simulink model "ABS_contDyn_model"  (R2022b)
settings: Solver=VariableStepAuto  StartTime=0.0  StopTime=tf  FixedStep=dt  MaxStep=dt  RelTol=1e-3
values from neighbouring files (symbols this model uses):
  hv = 0.3    [mainABS.m]
  init_speed = 100    [mainABS.m]
  lambda1_th = 0.2    [mainABS.m]
  lambda2_th = 0.1    [mainABS.m]
  omega_act = 70    [mainABS.m]
  omega_LPF = 100    [mainABS.m]
  rho = 0.9    [mainABS.m]
  rho_off = 0.9    [mainABS.m]
  rho_on = 1.1    [mainABS.m]
  tau_delay = 10e-3    (= 0.01)    [mainABS.m]
  Tb_dot_max = k    (= 5000)    [mainABS.m]
  Tb_max = 1500    [mainABS.m]
  v_on = 2.5    [mainABS.m]
  v_stop = 0.1    [mainABS.m]
undefined symbols (not defined in the file or in its folder): auxdata
libraries: simulink x2, dspsigops x1
settings Model: Creator=luca  LastModifiedBy=giacomo
settings SolverCC: AlgebraicLoopSolver=TrustRegion
settings DataIOCC: LimitDataPoints=on  ReturnWorkspaceOutputs=off
settings OptimizationCC: LifeSpan=inf
settings DebuggingCC: UnconnectedInputMsg=warning  UnconnectedOutputMsg=warning  UnconnectedLineMsg=warning  AllowSymbolicDim=off  SFUnexpectedBacktrackingDiag=warning  SFNoUnconditionalDefaultTransitionDiag=warning  SFExecutionAtInitializationDiag=none  SFMachineParentedDataDiag=warning  ArithmeticOperatorsInVariantConditions=warning
settings ModelReferenceCC: EnableRefExpFcnMdlSchedulingChecks=on  PropagateSignalLabelsOutOfModel=off
settings SFSimCC: SimUseLocalCustomCode=off  CustomCodeUndefinedFunction=UseInterfaceOnly
settings RTWCC: RTWUseLocalCustomCode=off
settings CodeAppCC: StateflowObjectComments=on
settings GRTTargetCC: TargetLangStandard=C89/C90 (ANSI)
settings ConfigComp: CovMetricSettings=dw  CovSaveCumulativeToWorkspaceVar=on  CovSaveSingleToWorkspaceVar=on  CovExternalEMLEnable=off

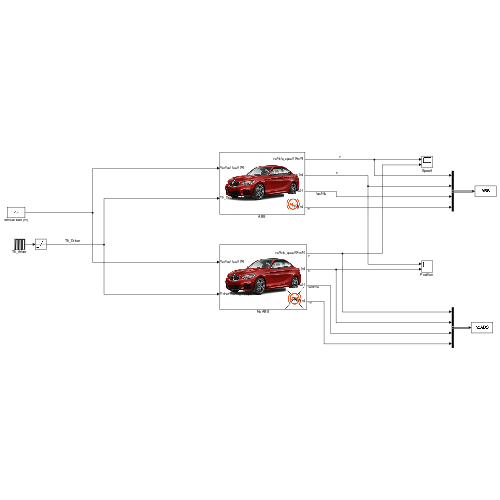
[thumbnail: Simulink's stored preview of the top-level diagram]
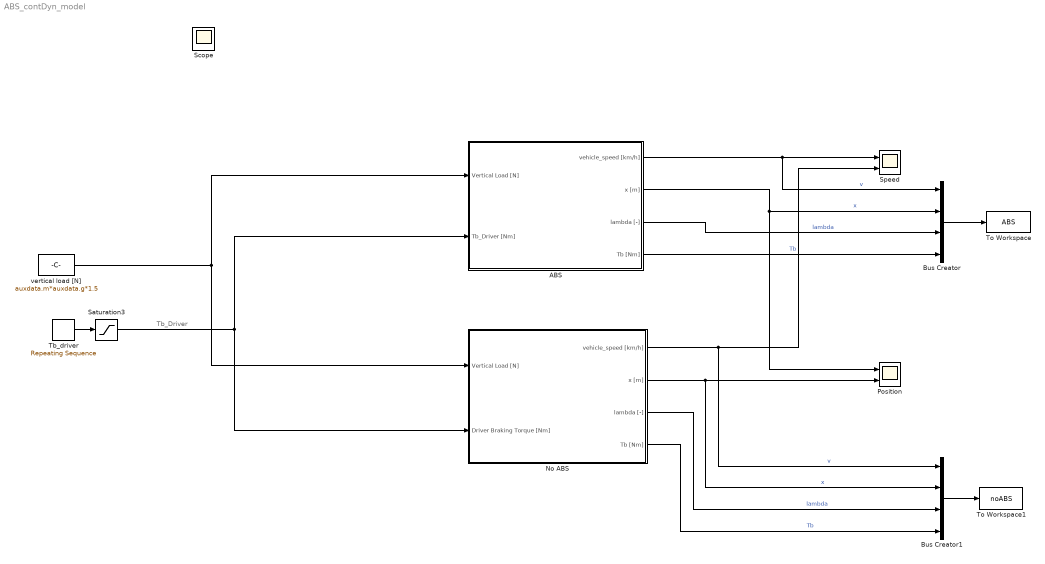
== system ABS_contDyn_model ==
  note: Tb_Driver
  ABS : Subsystem
      mask Display: image('figures/ABScar_on.png');
  Bus Creator : BusCreator  Inputs=4
  Bus Creator1 : BusCreator  Inputs=4
  No ABS : Subsystem
      mask Display: image('figures/ABS_off.png');
  Position : Scope  NumInputPorts=2
  Saturation3 : Saturate  UpperLimit=Tb_max  LowerLimit=0
  Speed : Scope  NumInputPorts=2
  Tb_driver : simulink/Sources/Repeating Sequence  rep_seq_t=time_manoeuvre  rep_seq_y=output_manoeuvre
  To Workspace : ToWorkspace  VariableName=ABS  SaveFormat=Timeseries  SampleTime=-1
  To Workspace1 : ToWorkspace  VariableName=noABS  SaveFormat=Timeseries  SampleTime=-1
  vertical load [N] : Constant  Value=auxdata.m*auxdata.g*1.5
  Scope : Scope
  wires:
  vertical load [N]/1 -> No ABS/1(Vertical Load [N]), ABS/1(Vertical Load [N])
  Saturation3/1 -> No ABS/2(Driver Braking Torque [Nm]), ABS/2(Tb_Driver [Nm])
  No ABS/1(" vehicle_speed [km/h]") -> Speed/2, Bus Creator1/1  "v"
  No ABS/2(x [m]) -> Position/2, Bus Creator1/2  "x"
  ABS/1(vehicle_speed [km/h]) -> Bus Creator/1, Speed/1  "v"
  ABS/2(x [m]) -> Position/1, Bus Creator/2  "x"
  Bus Creator/1 -> To Workspace/1
  ABS/3(lambda [-]) -> Bus Creator/3  "lambda"
  ABS/4(Tb [Nm]) -> Bus Creator/4  "Tb"
  Bus Creator1/1 -> To Workspace1/1
  No ABS/3(lambda [-]) -> Bus Creator1/3  "lambda"
  No ABS/4(Tb [Nm]) -> Bus Creator1/4  "Tb"
  Tb_driver/1 -> Saturation3/1

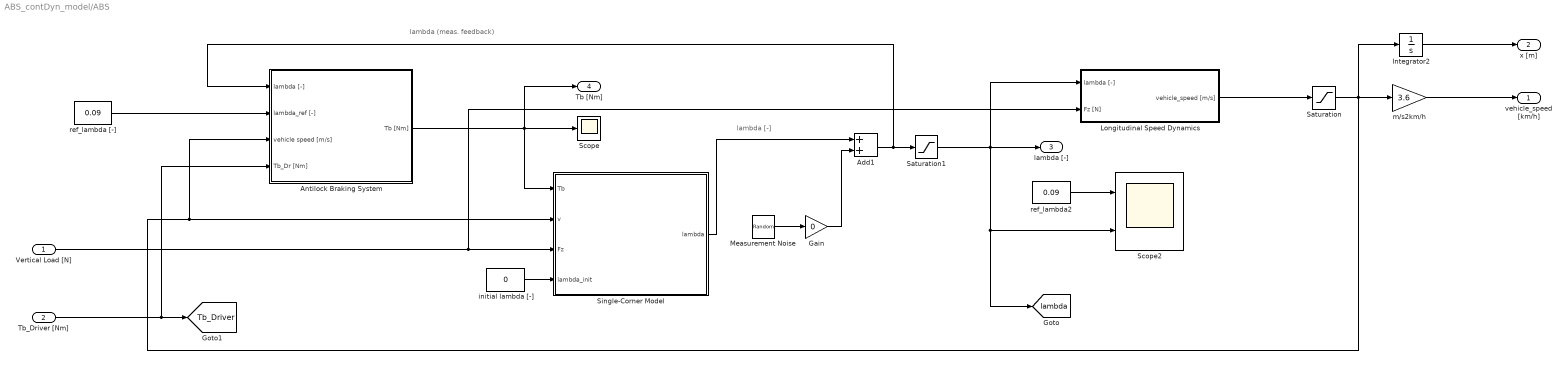
== system ABS_contDyn_model/ABS ==
  note: lambda [-]
  note: lambda (meas. feedback)
  Vertical Load [N] : Inport
  Tb_Driver [Nm] : Inport  Port=2
  Add1 : Sum
  Antilock Braking System : Subsystem
      mask Display: image('figures/ABS_on.png');
  Gain : Gain  Gain=0
  Integrator2 : Integrator
  Longitudinal Speed Dynamics : Subsystem
  Measurement Noise : RandomNumber  Variance=2e-5  SampleTime=0.001
  Saturation : Saturate  UpperLimit=100  LowerLimit=1e-3
  Saturation1 : Saturate  UpperLimit=1  LowerLimit=0
  Scope : Scope
  Scope2 : Scope  NumInputPorts=2
  Single-Corner Model : Subsystem
      mask Display:
      | image('figures/caliper_img.jpeg');
      | color('red');
      | port_label('output',1,'lambda');
      | port_label('input',1,'Tb');
      | port_label('input',2,'v');
      | port_label('input',3,'Fz');
      | port_label('input',4,'lambda_init');
  initial lambda [-] : Constant  Value=0
  m/s2km/h : Gain  Gain=3.6
  ref_lambda [-] : Constant  Value=0.09
  ref_lambda2 : Constant  Value=0.09
  vehicle_speed [km/h] : Outport
  x [m] : Outport  Port=2
  lambda [-] : Outport  Port=3
  Tb [Nm] : Outport  Port=4
  tag scope: Tb_Driver=global, lambda=global
  wires:
  m/s2km/h/1 -> vehicle_speed [km/h]/1
  Integrator2/1 -> x [m]/1
  Longitudinal Speed Dynamics/1(vehicle_speed [m/s]) -> Saturation/1
  Antilock Braking System/1(Tb [Nm]) -> Tb [Nm]/1, Single-Corner Model/1(Tb), Scope/1
  Saturation1/1 -> lambda [-]/1, Scope2/2, [lambda], Longitudinal Speed Dynamics/1(lambda [-])
  ref_lambda [-]/1 -> Antilock Braking System/2(lambda_ref [-])
  Gain/1 -> Add1/2
  Tb_Driver [Nm]/1 -> Antilock Braking System/4(Tb_Dr [Nm]), [Tb_Driver]
  Single-Corner Model/1(lambda) -> Add1/1
  Saturation/1 -> Integrator2/1, Single-Corner Model/2(v), Antilock Braking System/3(vehicle speed [m/s]), m/s2km/h/1
  Add1/1 -> Saturation1/1, Antilock Braking System/1(lambda [-])
  Measurement Noise/1 -> Gain/1
  Vertical Load [N]/1 -> Longitudinal Speed Dynamics/2(Fz [N]), Single-Corner Model/3(Fz)
  initial lambda [-]/1 -> Single-Corner Model/4(lambda_init)
  ref_lambda2/1 -> Scope2/1

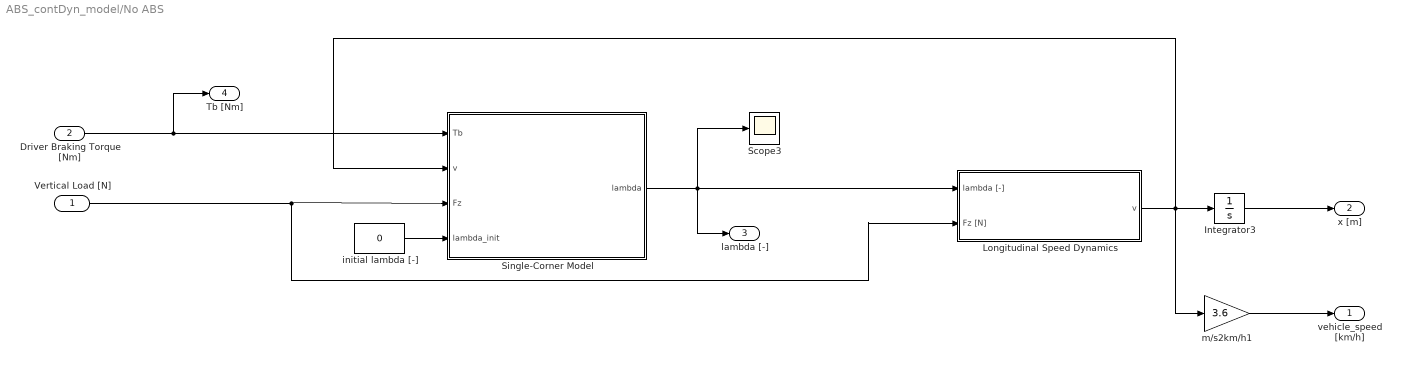
== system ABS_contDyn_model/No ABS ==
  Vertical Load [N] : Inport
  Driver Braking Torque [Nm] : Inport  Port=2
  Integrator3 : Integrator
  Longitudinal Speed Dynamics : Subsystem
  Scope3 : Scope
  Single-Corner Model : Subsystem
      mask Display:
      | image('figures/caliper_img.jpeg');
      | color('red');
      | port_label('output',1,'lambda');
      | port_label('input',1,'Tb');
      | port_label('input',2,'v');
      | port_label('input',3,'Fz');
      | port_label('input',4,'lambda_init');
  initial lambda [-] : Constant  Value=0
  m/s2km/h1 : Gain  Gain=3.6
  " vehicle_speed [km/h]" : Outport
  x [m] : Outport  Port=2
  lambda [-] : Outport  Port=3
  Tb [Nm] : Outport  Port=4
  wires:
  Single-Corner Model/1(lambda) -> lambda [-]/1, Longitudinal Speed Dynamics/1(lambda [-]), Scope3/1
  Vertical Load [N]/1 -> Longitudinal Speed Dynamics/2(Fz [N]), Single-Corner Model/3(Fz)
  Driver Braking Torque [Nm]/1 -> Tb [Nm]/1, Single-Corner Model/1(Tb)
  initial lambda [-]/1 -> Single-Corner Model/4(lambda_init)
  m/s2km/h1/1 -> " vehicle_speed [km/h]"/1
  Integrator3/1 -> x [m]/1
  Longitudinal Speed Dynamics/1(v) -> Integrator3/1, Single-Corner Model/2(v), m/s2km/h1/1

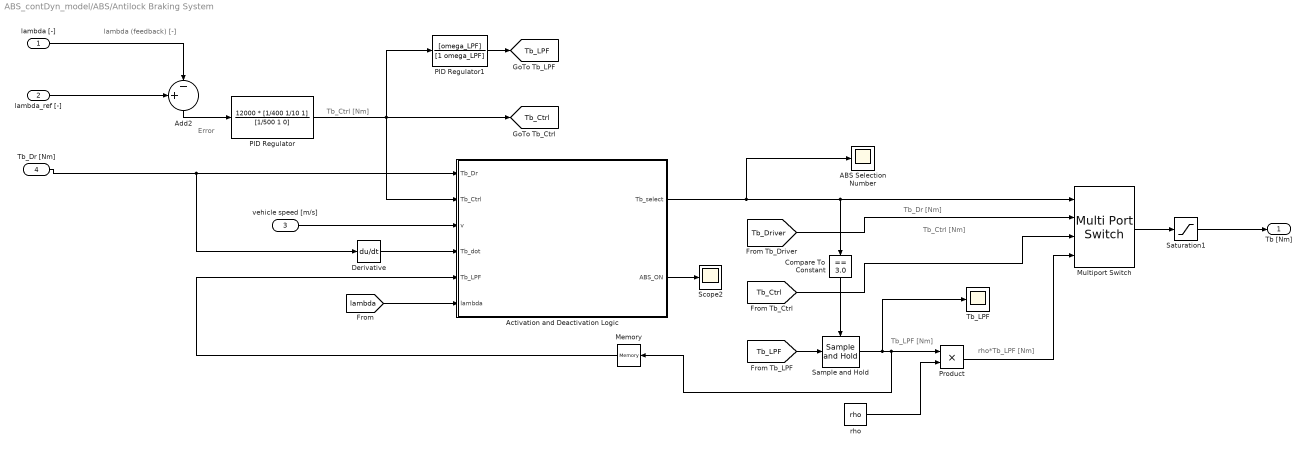
== system ABS_contDyn_model/ABS/Antilock Braking System ==
  note: Tb_LPF [Nm]
  note: Tb_Ctrl [Nm]
  note: Tb_Dr [Nm]
  note: lambda (feedback) [-]
  note: Error
  note: Tb_Ctrl [Nm]
  note: rho*Tb_LPF [Nm]
  lambda [-] : Inport
  lambda_ref [-] : Inport  Port=2
  vehicle speed [m/s] : Inport  Port=3
  Tb_Dr [Nm] : Inport  Port=4
  ABS Selection Number : Scope
  Activation and Deactivation Logic : Stateflow chart  TreatAsAtomicUnit=on
  Add2 : Sum  Inputs=+-|
  Compare To Constant : simulink/Logic and Bit Operations/Compare To Constant  relop===  const=3.0  OutDataTypeStr=boolean
  Derivative : Derivative
  Memory : Memory
  Multiport Switch : MultiPortSwitch  SaturateOnIntegerOverflow=off  InputSameDT=off
  PID Regulator : TransferFcn  Numerator=12000 * [1/400 1/10 1]  Denominator=[1/500 1 0]
  PID Regulator1 : TransferFcn  Numerator=[omega_LPF]  Denominator=[1 omega_LPF]
  Product : Product
  Sample and Hold : dspsigops/Sample and Hold  trig=Rising edge  initCond=0  latchinput=off
  Saturation1 : Saturate  UpperLimit=Tb_max  LowerLimit=0
  Scope2 : Scope
  Tb_LPF : Scope
  rho : Constant  Value=rho
  Tb [Nm] : Outport
  tag scope: Tb_Ctrl=global, Tb_LPF=global
  wires:
  lambda_ref [-]/1 -> Add2/1
  Activation and Deactivation Logic/2(ABS_ON) -> Scope2/1
  [Tb_Ctrl] -> Multiport Switch/3
  lambda [-]/1 -> Add2/2
  Tb_Dr [Nm]/1 -> Derivative/1, Activation and Deactivation Logic/1(Tb_Dr)
  vehicle speed [m/s]/1 -> Activation and Deactivation Logic/3(v)
  Multiport Switch/1 -> Saturation1/1
  Add2/1 -> PID Regulator/1
  [Tb_Driver] -> Multiport Switch/2
  Derivative/1 -> Activation and Deactivation Logic/4(Tb_dot)
  [lambda] -> Activation and Deactivation Logic/6(lambda)
  Activation and Deactivation Logic/1(Tb_select) -> ABS Selection Number/1, Multiport Switch/1, Compare To Constant/1
  Saturation1/1 -> Tb [Nm]/1
  PID Regulator/1 -> PID Regulator1/1, [Tb_Ctrl], Activation and Deactivation Logic/2(Tb_Ctrl)
  PID Regulator1/1 -> [Tb_LPF]
  [Tb_LPF] -> Sample and Hold/1
  Sample and Hold/1 -> Tb_LPF/1, Product/1, Memory/1
  Memory/1 -> Activation and Deactivation Logic/5(Tb_LPF)
  rho/1 -> Product/2
  Product/1 -> Multiport Switch/4
  Compare To Constant/1 -> Sample and Hold/Trigger

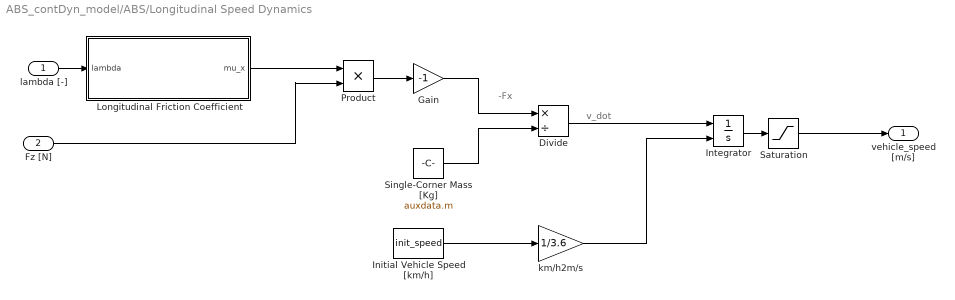
== system ABS_contDyn_model/ABS/Longitudinal Speed Dynamics ==
  note: -Fx
  note: v_dot
  lambda [-] : Inport
  Fz [N] : Inport  Port=2
  Divide : Product  Inputs=*/
  Gain : Gain  Gain=-1
  Initial Vehicle Speed [km/h] : Constant  Value=init_speed
  Integrator : Integrator  InitialConditionSource=external
  Longitudinal Friction Coefficient : MATLAB Function  TreatAsAtomicUnit=on
  Product : Product
  Saturation : Saturate  UpperLimit=100  LowerLimit=0
  Single-Corner Mass [Kg] : Constant  Value=auxdata.m
  km/h2m/s : Gain  Gain=1/3.6
  vehicle_speed [m/s] : Outport
  wires:
  Single-Corner Mass [Kg]/1 -> Divide/2
  Divide/1 -> Integrator/1
  km/h2m/s/1 -> Integrator/2
  Initial Vehicle Speed [km/h]/1 -> km/h2m/s/1
  Product/1 -> Gain/1
  Gain/1 -> Divide/1
  Saturation/1 -> vehicle_speed [m/s]/1
  Integrator/1 -> Saturation/1
  Longitudinal Friction Coefficient/1(mu_x) -> Product/1
  Fz [N]/1 -> Product/2
  lambda [-]/1 -> Longitudinal Friction Coefficient/1(lambda)

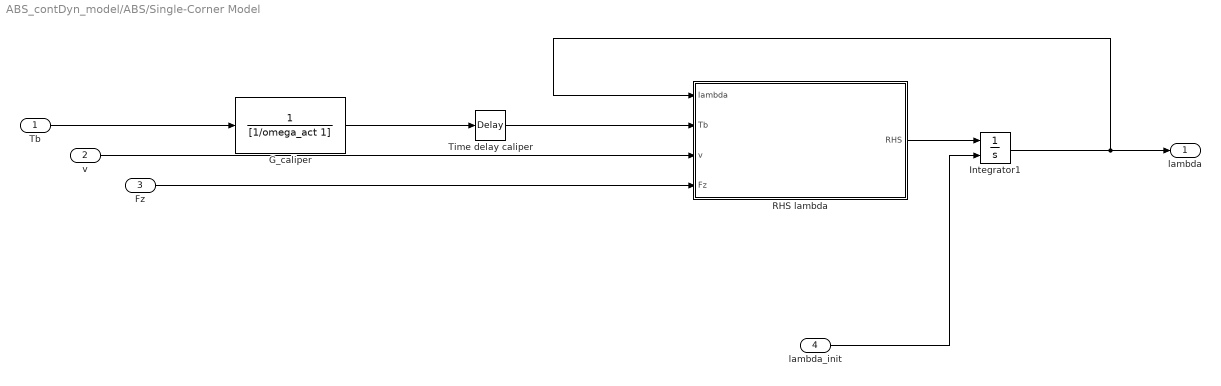
== system ABS_contDyn_model/ABS/Single-Corner Model ==
  Tb : Inport
  v : Inport  Port=2
  Fz : Inport  Port=3
  lambda_init : Inport  Port=4
  G_caliper : TransferFcn  Numerator=1  Denominator=[1/omega_act 1]
  Integrator1 : Integrator  InitialConditionSource=external
  RHS lambda : MATLAB Function  TreatAsAtomicUnit=on
  Time delay caliper : TransportDelay  DelayTime=tau_delay
  lambda : Outport
  wires:
  lambda_init/1 -> Integrator1/2
  RHS lambda/1(RHS) -> Integrator1/1
  v/1 -> RHS lambda/3(v)
  Fz/1 -> RHS lambda/4(Fz)
  Integrator1/1 -> RHS lambda/1(lambda), lambda/1
  G_caliper/1 -> Time delay caliper/1
  Time delay caliper/1 -> RHS lambda/2(Tb)
  Tb/1 -> G_caliper/1

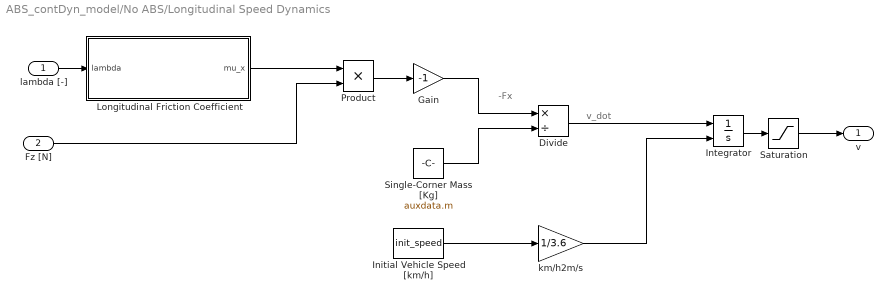
== system ABS_contDyn_model/No ABS/Longitudinal Speed Dynamics ==
  note: -Fx
  note: v_dot
  lambda [-] : Inport
  Fz [N] : Inport  Port=2
  Divide : Product  Inputs=*/
  Gain : Gain  Gain=-1
  Initial Vehicle Speed [km/h] : Constant  Value=init_speed
  Integrator : Integrator  InitialConditionSource=external
  Longitudinal Friction Coefficient : MATLAB Function  TreatAsAtomicUnit=on
  Product : Product
  Saturation : Saturate  UpperLimit=100  LowerLimit=1e-3
  Single-Corner Mass [Kg] : Constant  Value=auxdata.m
  km/h2m/s : Gain  Gain=1/3.6
  v : Outport
  wires:
  Single-Corner Mass [Kg]/1 -> Divide/2
  Divide/1 -> Integrator/1
  km/h2m/s/1 -> Integrator/2
  Initial Vehicle Speed [km/h]/1 -> km/h2m/s/1
  Product/1 -> Gain/1
  Gain/1 -> Divide/1
  Saturation/1 -> v/1
  Integrator/1 -> Saturation/1
  Longitudinal Friction Coefficient/1(mu_x) -> Product/1
  Fz [N]/1 -> Product/2
  lambda [-]/1 -> Longitudinal Friction Coefficient/1(lambda)

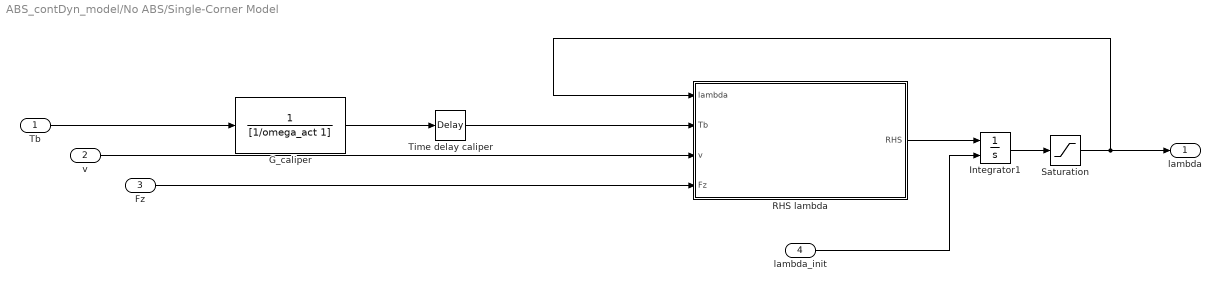
== system ABS_contDyn_model/No ABS/Single-Corner Model ==
  Tb : Inport
  v : Inport  Port=2
  Fz : Inport  Port=3
  lambda_init : Inport  Port=4
  G_caliper : TransferFcn  Numerator=1  Denominator=[1/omega_act 1]
  Integrator1 : Integrator  InitialConditionSource=external
  RHS lambda : MATLAB Function  TreatAsAtomicUnit=on
  Saturation : Saturate  UpperLimit=0.99  LowerLimit=0
  Time delay caliper : TransportDelay  DelayTime=tau_delay
  lambda : Outport
  wires:
  lambda_init/1 -> Integrator1/2
  RHS lambda/1(RHS) -> Integrator1/1
  v/1 -> RHS lambda/3(v)
  Fz/1 -> RHS lambda/4(Fz)
  Integrator1/1 -> Saturation/1
  G_caliper/1 -> Time delay caliper/1
  Time delay caliper/1 -> RHS lambda/2(Tb)
  Tb/1 -> G_caliper/1
  Saturation/1 -> RHS lambda/1(lambda), lambda/1

== matlab function ABS_contDyn_model/ABS/Single-Corner Model/RHS lambda ==
  data: lambda input; RHS output; Tb input; v input; Fz input; auxdata parameter
function RHS = lambdaDyn( lambda, Tb, v, Fz, auxdata )
% Right hand side of the longitudinal slip dynamics

omega = (1 - lambda) * v / auxdata.r_w;

% Equilibrium manifold
%        /      (1 - lambda) * J \
% Psi = | r_w + ----------------  | * Fz * mu
%        \          r_w * m      /
Psi = (auxdata.r_w + ...
       auxdata.J / (auxdata.r_w * auxdata.m) * (1 - lambda)) * Fz * ...
       burckhardt( lambda, auxdata.road_condition );

if omega <= 0.1
    RHS = 0;
else
    RHS = -(1 - lambda) / (auxdata.J * omega) * (Psi - Tb);
end

end

== matlab function ABS_contDyn_model/ABS/Longitudinal Speed Dynamics/Longitudinal Friction Coefficient ==
  data: lambda input; mu_x output; auxdata parameter
function mu_x = LongitudinalFrction(lambda,auxdata)
    
mu_x = burckhardt(lambda,auxdata.road_condition);

end

== matlab function ABS_contDyn_model/No ABS/Single-Corner Model/RHS lambda ==
  data: lambda input; RHS output; Tb input; v input; Fz input; auxdata parameter
function RHS = lambdaDyn( lambda, Tb, v, Fz, auxdata )
% Right hand side of the longitudinal slip dynamics

omega = (1 - lambda) * v / auxdata.r_w;

% Equilibrium manifold
%        /      (1 - lambda) * J \
% Psi = | r_w + ----------------  | * Fz * mu
%        \          r_w * m      /
Psi = (auxdata.r_w + ...
       auxdata.J / (auxdata.r_w * auxdata.m) * (1 - lambda)) * Fz * ...
       burckhardt( lambda, auxdata.road_condition );

if omega <= 0.1
    RHS = 0;
else
    RHS = -(1 - lambda) / (auxdata.J * omega) * (Psi - Tb);
end

end

== matlab function ABS_contDyn_model/No ABS/Longitudinal Speed Dynamics/Longitudinal Friction Coefficient ==
  data: lambda input; mu_x output; auxdata parameter
function mu_x = LongitudinalFrction( lambda, auxdata )
    
mu_x = burckhardt( lambda, auxdata.road_condition );

end

== stateflow chart ABS_contDyn_model/ABS/Antilock Braking System/Activation and Deactivation Logic ==
  state abs_OFF
    ABS_ON = 0;
    state High_Speed_OFF
      Tb_select = 1;
    state Low_Speed_OFF
      Tb_select = 1;
    (default) -> High_Speed_OFF
    High_Speed_OFF -> Low_Speed_OFF [order 2] : [v < v_on - hv]
    Low_Speed_OFF -> High_Speed_OFF : [v > v_on + hv]
  state abs_ON
    ABS_ON = 1;
    state High_Speed_ON
      Tb_select = 2;
    state Low_Speed_ON
      Tb_select = 3;
    High_Speed_ON -> Low_Speed_ON [order 2] : [v < v_on]
  (default) -> abs_OFF
  High_Speed_OFF -> High_Speed_ON [order 1] : [v > v_on && ...
      | Tb_Dr > rho_on * Tb_Ctrl && ...
      | lambda > lambda1_th - (((lambda1_th - lambda2_th) * Tb_dot) / Tb_dot_max) ]
  High_Speed_ON -> High_Speed_OFF [order 1] : [Tb_Dr < rho_off * Tb_Ctrl]
  Low_Speed_ON -> Low_Speed_OFF : [v < v_stop || ...
      | Tb_Dr < rho_off * Tb_LPF]
  data: Tb_select output; Tb_Dr input; Tb_Ctrl input; v input; Tb_dot input; Tb_dot_max parameter; v_on parameter; rho_on parameter; Tb_LPF input; lambda input; lambda1_th parameter; v_stop parameter; hv parameter; rho_off parameter; ABS_ON output; lambda2_th parameter
